simulink model "Linear_Kalman"  (R2021a)
settings: Solver=VariableStepAuto  StartTime=0.0  StopTime=10.0  RelTol=1e-3
values from neighbouring files (symbols this model uses):
  A = [0 1;(-g/l) 0]    [Inverted_Pen.m]
  B = [0;1/(m*l^2)]    [Inverted_Pen.m]
  C = [1 0]    [Inverted_Pen.m]
  D = 0    [Inverted_Pen.m]
  g = 9.81    [Inverted_Pen.m]
  l = 2.5    [Inverted_Pen.m]
  m = 2    [Inverted_Pen.m]
  Q = 2e-4    (= 0.0002)    [Inverted_Pen.m]
  R = 2e-4    (= 0.0002)    [Inverted_Pen.m]
  Ts = 0.01    [Inverted_Pen.m]
  x_0 = [pi/18 0]    [Inverted_Pen.m]
undefined symbols (not defined in the file or in its folder): Continuous, Time
libraries: simulink x2, ctrlSharedLib x1
settings Model: Creator=SOLONSO  LastModifiedBy=SOLONSO

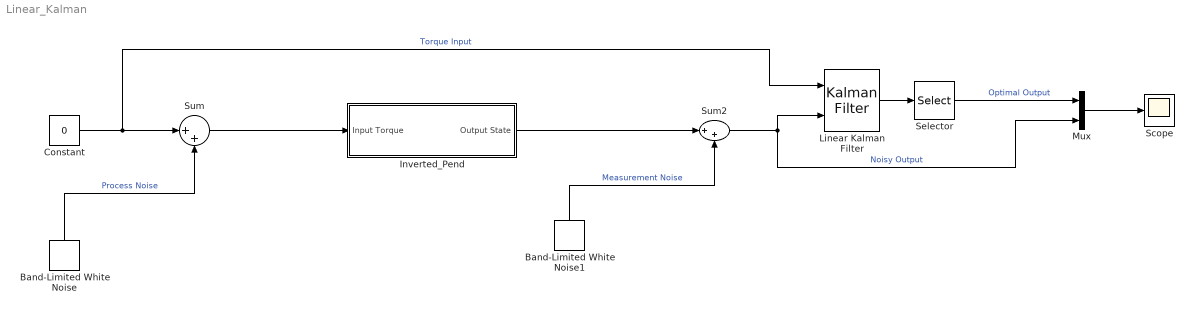
== system Linear_Kalman ==
  Band-Limited White Noise : simulink/Sources/Band-Limited White Noise  Cov=Q*Ts  Ts=Ts  seed=[23341]
  Band-Limited White Noise1 : simulink/Sources/Band-Limited White Noise  Cov=R*Ts  Ts=Ts  seed=[23391]
  Constant : Constant  Value=0
  Inverted_Pend : Subsystem
  Linear Kalman Filter : ctrlSharedLib/Kalman Filter  TimeDomain=Continuous-Time  UseCurrentEstimator=on  ModelSource=Individual A, B, C, D matrices  ModelSourceVariable=ss(0.95,1,1,0,1)  A=A  B=B  C=C  D=D  NumberOfStates=1  NumberOfInputs=1  NumberOfOutputs=1  InitialEstimateSource=Dialog  X0=x_0  P0=10  UseK=off  UseGH=off  NumberOfProcessNoiseInputs=1  G=1  TimeInvariantG=on  H=0  TimeInvariantH=on  Q=diag([0 Q])  TimeInvariantQ=on  R=R  TimeInvariantR=on  N=0  TimeInvariantN=on  AddInputPort=on  AddEnablePort=off  OutputEstimatedY=off  OutputP=off  Ts=-1
  Mux : Mux  Inputs=2
  Scope : Scope
  Selector : Selector  InputPortWidth=2  IndexOptions=Index vector (dialog)  Indices=1  OutputSizes=1
  Sum : Sum  Inputs=|++
  Sum2 : Sum  Inputs=|++
  wires:
  Sum2/1 -> Linear Kalman Filter/2, Mux/2  "Noisy Output"
  Linear Kalman Filter/1 -> Selector/1
  Band-Limited White Noise/1 -> Sum/2  "Process Noise"
  Band-Limited White Noise1/1 -> Sum2/2  "Measurement Noise"
  Selector/1 -> Mux/1  "Optimal Output"
  Constant/1 -> Linear Kalman Filter/1, Sum/1  "Torque Input"
  Mux/1 -> Scope/1
  Sum/1 -> Inverted_Pend/1(Input Torque)
  Inverted_Pend/1(Output State) -> Sum2/1

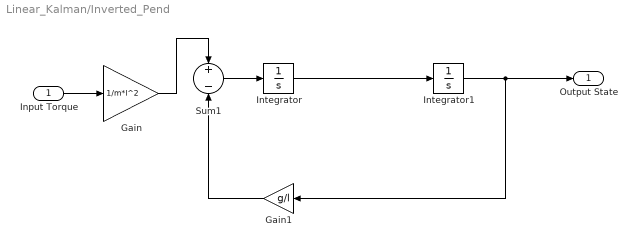
== system Linear_Kalman/Inverted_Pend ==
  Input Torque : Inport
  Gain : Gain  Gain=1/m*l^2
  Gain1 : Gain  Gain=g/l
  Integrator : Integrator
  Integrator1 : Integrator  InitialCondition=pi/18
  Sum1 : Sum  Inputs=+-
  Output State : Outport
  wires:
  Sum1/1 -> Integrator/1
  Integrator1/1 -> Output State/1, Gain1/1
  Gain1/1 -> Sum1/2
  Integrator/1 -> Integrator1/1
  Gain/1 -> Sum1/1
  Input Torque/1 -> Gain/1
